simulink model "ABS"  (R2015a)
settings: Solver=ode45  StartTime=0.0  StopTime=10.0  RelTol=1e-3
settings Model: Creator=Teme  LastModifiedBy=Teme
settings RTWCC: Toolchain=Clang v3.1 | gmake (64-bit Mac)

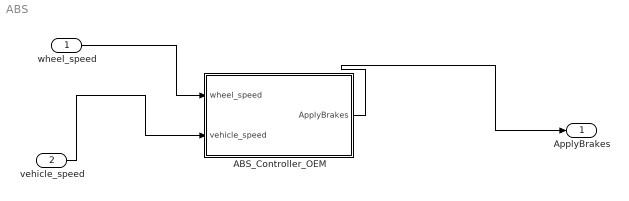
== system ABS ==
  wheel_speed : Inport  SampleTime=0
  vehicle_speed : Inport  Port=2  SampleTime=0
  ABS_Controller_OEM : Subsystem
  ApplyBrakes : Outport
  wires:
  wheel_speed/1 -> ABS_Controller_OEM/1(wheel_speed)
  vehicle_speed/1 -> ABS_Controller_OEM/2(vehicle_speed)
  ABS_Controller_OEM/1(ApplyBrakes) -> ApplyBrakes/1

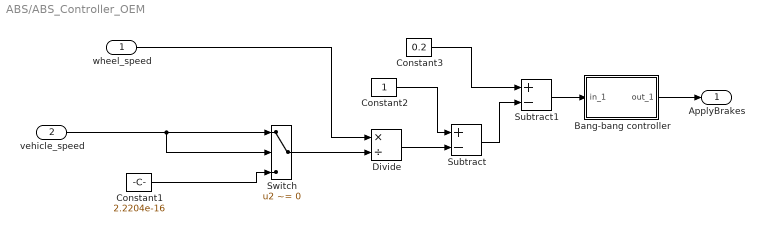
== system ABS/ABS_Controller_OEM ==
  wheel_speed : Inport  SampleTime=0
  vehicle_speed : Inport  Port=2  SampleTime=0
  Bang-bang controller : Subsystem  mask(Sign){}
      mask help: y = sign(x)
      mask Help: Sign Function:\n\t\t\ty = 1 if x > 0\n\t\t\ty = 0 if x = 0\n\t\t\ty = -1 if x < 0
      mask Display: plot(-50,-50,50,50,[-50,50],[0,0],[0,0],[-50,50],[-40,0],[-30,-30],[0,40],[30,30])
  Constant1 : Constant  RequirementInfo={} %GIDa_68c76990_35e6_402e_a499_fea0c7d912d5  Value=2.2204e-16  VectorParams1D=off
  Constant2 : Constant  RequirementInfo={} %GIDa_4a8a2e2c_8a4d_462f_a92b_c4449d5218d4  VectorParams1D=off
  Constant3 : Constant  RequirementInfo={} %GIDa_3f3dfe3e_fba3_4463_89e1_4e0ea70d5db5  Value=0.2  VectorParams1D=off
  Divide : Product  Inputs=*/
  Subtract : Sum  Inputs=+-
  Subtract1 : Sum  Inputs=+-
  Switch : Switch  RequirementInfo={} %GIDa_2bb70abf_1eef_45bd_b310_739057b34ef7  Criteria=u2 ~= 0
  ApplyBrakes : Outport
  wires:
  wheel_speed/1 -> Divide/1
  Constant1/1 -> Switch/3
  Divide/1 -> Subtract/2
  Constant2/1 -> Subtract/1
  Switch/1 -> Divide/2
  vehicle_speed/1 -> Switch/2, Switch/1
  Constant3/1 -> Subtract1/1
  Subtract1/1 -> Bang-bang controller/1(in_1)
  Bang-bang controller/1(out_1) -> ApplyBrakes/1
  Subtract/1 -> Subtract1/2

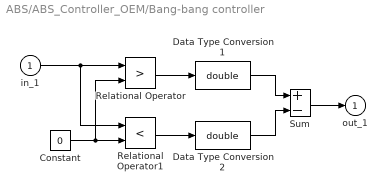
== system ABS/ABS_Controller_OEM/Bang-bang controller ==
  in_1 : Inport
  Constant : Constant  Value=0
  Data Type Conversion1 : DataTypeConversion  OutDataTypeStr=double  SaturateOnIntegerOverflow=on  RndMeth=Zero
  Data Type Conversion2 : DataTypeConversion  OutDataTypeStr=double  SaturateOnIntegerOverflow=on  RndMeth=Zero
  Relational Operator : RelationalOperator  Operator=>  OutDataTypeStr=boolean  InputSameDT=on
  Relational Operator1 : RelationalOperator  Operator=<  OutDataTypeStr=boolean  InputSameDT=on
  Sum : Sum  Inputs=+-  SaturateOnIntegerOverflow=on  InputSameDT=on  OutDataTypeStr=Inherit: Same as first input
  out_1 : Outport  InitialOutput=0
  wires:
  Data Type Conversion2/1 -> Sum/2
  Data Type Conversion1/1 -> Sum/1
  Sum/1 -> out_1/1
  Relational Operator/1 -> Data Type Conversion1/1
  Relational Operator1/1 -> Data Type Conversion2/1
  Constant/1 -> Relational Operator/2, Relational Operator1/2
  in_1/1 -> Relational Operator1/1, Relational Operator/1
